simulink model "jsbsim_trim_mod"  (Simulink 7.5)
settings: Solver=ode3  StartTime=0.0  StopTime=JSBSimTrim.FinalTime  FixedStep=JSBSimTrim.SampleTime  RelTol=1e-3
undefined symbols (not defined in the file or in its folder): JSBSimTrim
settings Model: Creator=Bri  LastModifiedBy=biffbutkus
settings DataIOCC: SaveOutput=off  SaveTime=off
settings DebuggingCC: SolverPrmCheckMsg=none  UnconnectedInputMsg=none  UnconnectedOutputMsg=none  UnconnectedLineMsg=none  StrictBusMsg=Warning

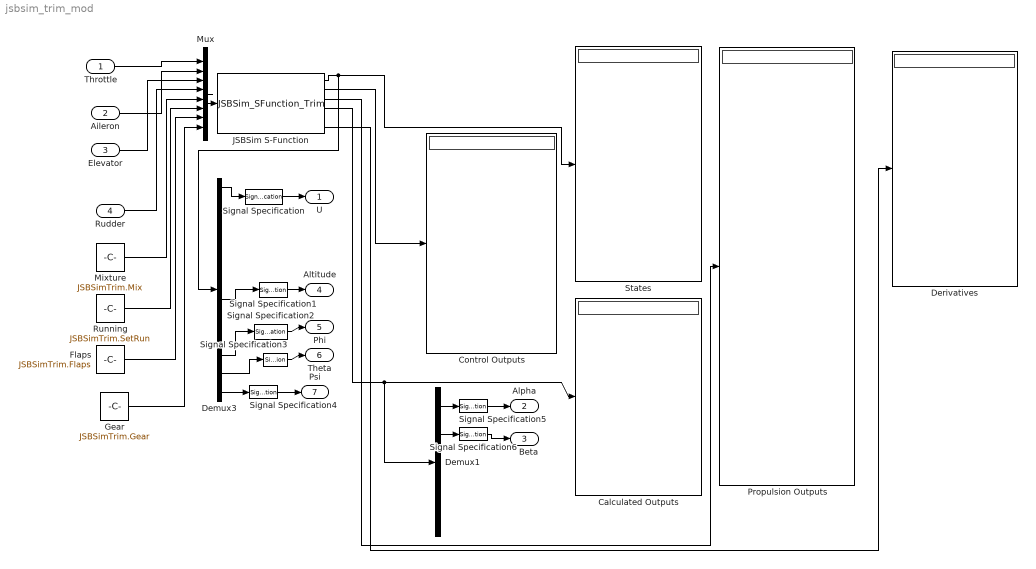
== system jsbsim_trim_mod ==
  Throttle : Inport  PortDimensions=1  OutDataType=sfix(16)  OutScaling=2^0
  Aileron : Inport  Port=2  PortDimensions=1  OutDataType=sfix(16)  OutScaling=2^0
  Elevator : Inport  Port=3  PortDimensions=1  OutDataType=sfix(16)  OutScaling=2^0
  Rudder : Inport  Port=4  PortDimensions=1  OutDataType=sfix(16)  OutScaling=2^0
  Calculated Outputs : Display
  Control Outputs : Display
  Demux1 : Demux  Outputs=11
  Demux3 : Demux  Outputs=12
  Derivatives : Display
  Flaps : Constant  Value=JSBSimTrim.Flaps  OutDataType=sfix(16)  OutScaling=2^0
  Gear : Constant  Value=JSBSimTrim.Gear  OutDataType=sfix(16)  OutScaling=2^0
  JSBSim S-Function : S-Function  FunctionName=JSBSim_SFunction_Trim  Parameters=ac_name, IC_states, IC_controls, IC_delta_t, IC_verbosity,IC_sim_multiplier, IC_solver,IC_fv_sim, IC_fv_trim  EnableBusSupport=off  mask{ac_name=JSBSimTrim.Aircraft, IC_states=JSBSimTrim.ICStates, IC_controls=JSBSimTrim.ICInputs, IC_delta_t=JSBSimTrim.SampleTime, IC_verbosity=JSBSimTrim.Verbosity, IC_sim_multiplier=1, IC_solver=0, IC_fv_sim=0, IC_fv_trim=JSBSimTrim.FlightViz}
      mask prompts: ac_name "AC:"; IC_states "States:"; IC_controls "Controls:"; IC_delta_t "Delta:"; IC_verbosity "Verbosity:"; IC_sim_multiplier "JSBSim Multiplier:"; IC_solver "JSBSim Solvers"; IC_fv_sim "FlightViz sim"; IC_fv_trim "FlightViz trim"
  Mixture : Constant  Value=JSBSimTrim.Mix  OutDataType=sfix(16)  OutScaling=2^0
  Mux : Mux  Inputs=8
  Propulsion Outputs : Display
  Running : Constant  Value=JSBSimTrim.SetRun  OutDataType=sfix(16)  OutScaling=2^0
  Signal Specification{,1..6} (7 alike) : SignalSpecification  Dimensions=1  DataType=double  OutDataType=sfix(16)  OutScaling=2^0  OutDataTypeStr=double
  States : Display
  U : Outport  OutDataType=sfix(16)  OutScaling=2^0
  Alpha : Outport  Port=2  OutDataType=sfix(16)  OutScaling=2^0
  Beta : Outport  Port=3  OutDataType=sfix(16)  OutScaling=2^0
  Altitude : Outport  Port=4  OutDataType=sfix(16)  OutScaling=2^0
  Phi : Outport  Port=5  OutDataType=sfix(16)  OutScaling=2^0
  Theta : Outport  Port=6  OutDataType=sfix(16)  OutScaling=2^0
  Psi : Outport  Port=7  OutDataType=sfix(16)  OutScaling=2^0
  wires:
  JSBSim S-Function/1 -> States/1, Demux3/1
  Mux/1 -> JSBSim S-Function/1
  Throttle/1 -> Mux/1
  Aileron/1 -> Mux/2
  Elevator/1 -> Mux/3
  Rudder/1 -> Mux/4
  Mixture/1 -> Mux/5
  Running/1 -> Mux/6
  Flaps/1 -> Mux/7
  Gear/1 -> Mux/8
  JSBSim S-Function/2 -> Control Outputs/1
  JSBSim S-Function/3 -> Propulsion Outputs/1
  JSBSim S-Function/4 -> Calculated Outputs/1, Demux1/1
  Demux3/1 -> Signal Specification/1
  Demux1/2 -> Signal Specification5/1
  Demux1/4 -> Signal Specification6/1
  Demux3/7 -> Signal Specification1/1
  Demux3/10 -> Signal Specification2/1
  Demux3/11 -> Signal Specification3/1
  Demux3/12 -> Signal Specification4/1
  Signal Specification/1 -> U/1
  Signal Specification1/1 -> Altitude/1
  Signal Specification2/1 -> Phi/1
  Signal Specification3/1 -> Theta/1
  Signal Specification4/1 -> Psi/1
  Signal Specification5/1 -> Alpha/1
  Signal Specification6/1 -> Beta/1
  JSBSim S-Function/6 -> Derivatives/1
